simulink model "uz_mpc_6ph_sca"  (R2022b)
settings: Solver=FixedStepDiscrete  StartTime=0.0  StopTime=ST  RelTol=1e-3
InitFcn:
  | clear
  | clc
  | 
  | f_clock = 100e6;        % IP core clock freq in Hz
  | t_clock = 1/f_clock;    % IP core sample time in s
  | 
  | f_ADC =100e3;           % ADC interrupt freq in Hz
  | t_ADC = 1/f_ADC;        % ADC sample time in s
  | Ts = t_ADC;
  | 
  | % amplitude of sinusoidal signal sources
  | A = 0.1;
  | 
  | % machine parameters
  | Rs = 0.27;              % Phase resistance in Ohm
  | psi_pm = 0.19;          % PM flux linkage in Vs
  | Ld = 1.7e-3;            % d-inductance in H
  | Lq = 3.8e-3;            % q-inductance in H
  | Lx = 2.4e-3;            % x-inductance in H
  | Ly = 2.5e-3;            % y-inductance in H
  | p = 5;                  % pole pairs
  | 
  | VR = 400;               % Rated eff. line-line voltage in V
  | IR = 10/sqrt(2);             % Rated eff. phase current in A
  | % IR = 14.142;
  | nR = 3000;              % Rated mechanical speed in 1/min
  | 
  | % p.u. base units acc. to T.Geyer, Model predictive control of high power
  | % converters and industrial drives. Hoboken, NJ, USA: Wiley, 2016, Chapter 2.1.2
  | VB = sqrt(2/3)*VR;
  | IB = sqrt(2)*IR;
  | omegaB = nR*2*pi()/60*p;
  | ZB = VB/IB;
  | LB = ZB/omegaB;
  | SB = 3/2 *VB*IB;
  | psiB = VB/omegaB;
  | TB = psiB*IB;
  | 
  | %pre calculated constants - check results regarding fixd_type_constants!!!
  | Rs_over_ZB = Rs/ZB;
  | Ts_times_ZB_over_Ld = Ts*ZB/Ld;
  | Ts_times_ZB_over_Lq = Ts*ZB/Lq;
  | Ts_times_ZB_over_Lx = Ts*ZB/Lx;
  | Ts_times_ZB_over_Ly = Ts*ZB/Ly;
  | Ld_over_LB = Ld/LB;
  | Lq_over_LB = Lq/LB;
  | Ld_minus_Lq_over_LB = (Ld-Lq)/LB;
  | psi_pm_over_psiB = psi_pm/psiB;
  | 
  | % fixed-point data types
  | pu_fixdt_type = fixdt(1,18,15); % output data type of pu values
  | % fixdt_type_dq_currents = fixdt(1,27,16);
  | fixdt_type_dq_currents = fixdt(1,27,24);
  | fixdt_type_xy_currents = fixdt(1,18,11);
  | fixdt_type_dqxy_ref_currents = fixdt(1,18,15);
  | fixdt_type_dqxy_voltages = fixdt(1,27,24);
  | fixdt_type_angle = fixdt(1,24,20);
  | % fixdt_type_sin_cos = fixdt(1,18,16);
  | fixdt_type_sin_cos = fixdt(1,27,20);
  | fixdt_type_lambda = fixdt(0,18,17);
  | ... (+38 lines)
libraries: nesl_utility x44, fl_lib x41, simulink x23, ee_lib x12, hdlsllib x2, spsAlphaBetaZerotodq0Lib x1, batteryecm_lib x1
(part 2 of 4)

== system uz_mpc_6ph_sca/counter_f_sw_6ph ==
  note: To avoid unneccessary calcualtions, i divide by 24 on the ARM processor.
  note: Over AXI, 32 Bit are received.
      | However, only one Bit is used.
  note: 1 for one cycle if edge recognized
  note: Since i count now every On and Off Transition for each switch,
      |  i have to divide by 12*2 in order to get the switching frequency
      |  (after dividing by the time).
      | 12 comes from the 12 switches
      | 2 comes from that 1 ON-transition and 1 OFF-transition = 1 switching-cycle
  ss_in_0 : Inport
  ss_in_1 : Inport  Port=2
  ss_in_2 : Inport  Port=3
  ss_in_3 : Inport  Port=4
  ss_in_4 : Inport  Port=5
  ss_in_5 : Inport  Port=6
  ss_in_6 : Inport  Port=7
  ss_in_7 : Inport  Port=8
  ss_in_8 : Inport  Port=9
  ss_in_9 : Inport  Port=10
  ss_in_10 : Inport  Port=11
  ss_in_11 : Inport  Port=12
  bResetAXI : Inport  Port=13
  Count_f_sw : MATLAB Function  TreatAsAtomicUnit=on  VariantControl=(default)
  Detec_edge : Sum  Inputs=+-  AccumDataTypeStr=int8  OutDataTypeStr=int8
  Gain : Gain  Commented=on  Gain=1/(12*2)
  Mux : Mux  Inputs=6
  Mux1 : Mux  Inputs=6
  Mux2 : Mux  Inputs=2
  SS_Old : Delay  DelayLength=1
  Saturation : Saturate  UpperLimit=1  LowerLimit=0  OutMin=[0]  OutMax=[1]  OutDataTypeStr=fixdt(0,1)
  Scope : Scope  NumInputPorts=2
  delay : Delay  DelayLength=1
  reset_old2 : Delay  DelayLength=1
  reset_old_switch1 : Switch  Criteria=u2 ~= 0  SaturateOnIntegerOverflow=off  InputSameDT=off
  switchNumb_AXI : Outport  VectorParamsAs1DForOutWhenUnconnected=off
  switchNumb : Outport  Port=2  VectorParamsAs1DForOutWhenUnconnected=off
  wires:
  ss_in_9/1 -> Mux1/4
  ss_in_6/1 -> Mux1/1
  ss_in_10/1 -> Mux1/5
  ss_in_11/1 -> Mux1/6
  ss_in_8/1 -> Mux1/3
  ss_in_1/1 -> Mux/2
  ss_in_5/1 -> Mux/6
  Saturation/1 -> Count_f_sw/4(bReset), Scope/1
  ss_in_4/1 -> Mux/5
  Mux/1 -> Mux2/1
  ss_in_2/1 -> Mux/3
  ss_in_0/1 -> Mux/1
  Mux2/1 -> SS_Old/1, Count_f_sw/3(ss_v)
  delay/1 -> Count_f_sw/1(switchNumb)
  reset_old2/1 -> Detec_edge/2, reset_old_switch1/3
  Detec_edge/1 -> Saturation/1, reset_old_switch1/2  "1 for one cycle if edge recognized"
  Mux1/1 -> Mux2/2
  reset_old_switch1/1 -> reset_old2/1
  ss_in_7/1 -> Mux1/2
  bResetAXI/1 -> Scope/2, reset_old_switch1/1, Detec_edge/1
  ss_in_3/1 -> Mux/4
  SS_Old/1 -> Count_f_sw/2(ss_v_old)
  Count_f_sw/1(switchNumbOut) -> delay/1, switchNumb_AXI/1, switchNumb/1

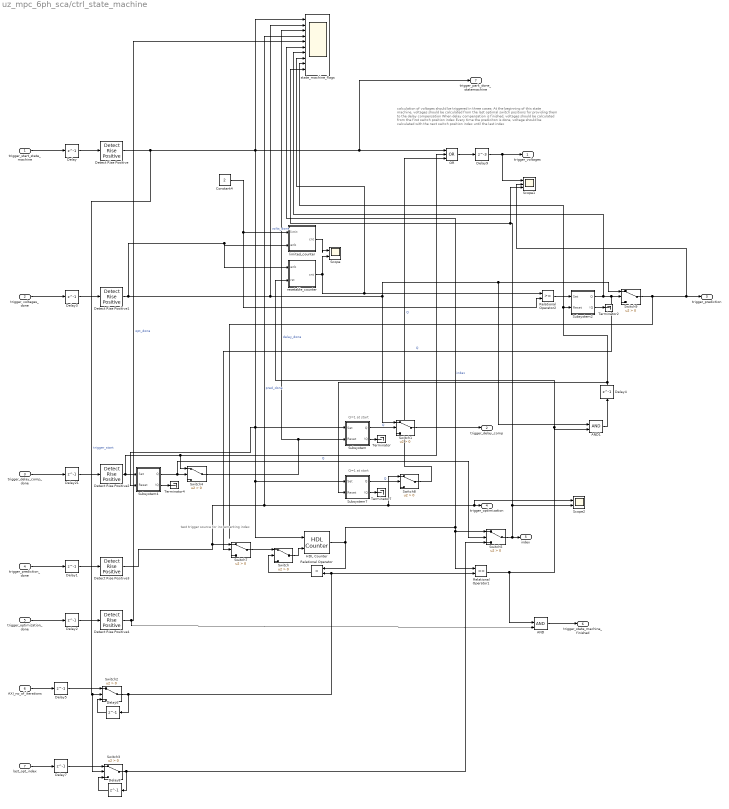
== system uz_mpc_6ph_sca/ctrl_state_machine ==
  note: test trigger source for incrementing index
  note: calculation of voltages should be triggered in three cases:
      |
      | At the beginning of this state machine, voltages should be calculated from the last optimal switch positions for providing them to the delay compensation
      | When delay compensation is finished, voltages should be calculated from the first switch position index
      | Every time the prediciton is done, voltage should be calculated with the next switch position index until the last index
  note: Q=1 at start
  note: Q=1 at start
  trigger_start_state_machine : Inport
  trigger_voltages_done : Inport  Port=2
  trigger_delay_comp_done : Inport  Port=3
  trigger_prediction_done : Inport  Port=4
  trigger_optimization_done : Inport  Port=5
  AXI_no_of_iterations : Inport  Port=6  OutDataTypeStr=uint32
  last_opt_index : Inport  Port=7  OutDataTypeStr=uint32
  AND : Logic  IconShape=distinctive  AllPortsSameDT=off  OutDataTypeStr=boolean
  AND1 : Logic  IconShape=distinctive  AllPortsSameDT=off  OutDataTypeStr=boolean
  Constant4 : Constant  Value=2  OutDataTypeStr=uint8  SampleTime=-1
  Delay{,1..8,21} (10 alike) : Delay  DelayLength=1
  Delay9 : Delay  DelayLength=3
  Detect Rise Positive{,1..4} (5 alike) : simulink/Logic and Bit Operations/Detect Rise Positive  vinit=0  OutDataTypeStr=boolean
  HDL Counter : hdlsllib/Sources/HDL Counter  CountType=Free running  CountInit=1  CountStep=1  CountMax=25  CountFromType=Initial value  CountFrom=1  CountResetPort=on  CountLoadPort=off  CountEnbPort=on  CountDirPort=off  CountHitOutputPort=off  CountDataType=Unsigned  CountWordLen=32  CountFracLen=0  CountSampTime=1
  OR : Logic  Operator=OR  Inputs=3  IconShape=distinctive  AllPortsSameDT=off  OutDataTypeStr=boolean
  Relational Operator : RelationalOperator  Operator=<  OutDataTypeStr=boolean  RndMeth=Simplest  InputSameDT=off
  Relational Operator1 : RelationalOperator  Operator===  OutDataTypeStr=boolean  RndMeth=Simplest  InputSameDT=off
  Relational Operator2 : RelationalOperator  OutDataTypeStr=boolean  RndMeth=Simplest  InputSameDT=off
  Scope : Scope  NumInputPorts=2
  Scope1 : Scope  NumInputPorts=3
  Scope2 : Scope  NumInputPorts=2
  Subsystem : Subsystem
  Subsystem2 : Subsystem
  Subsystem4 : Subsystem
  Subsystem7 : Subsystem
  Switch{,1..5,7..9} (9 alike) : Switch  Criteria=u2 > Threshold  SaturateOnIntegerOverflow=off  InputSameDT=off
  Terminator{,2,4,7} (4 alike) : Terminator
  limited_counter : Subsystem
  resetable_counter : Subsystem
  state_machine_flags : Scope  NumInputPorts=10
  trigger_voltages : Outport  VectorParamsAs1DForOutWhenUnconnected=off
  trigger_delay_comp : Outport  Port=2  VectorParamsAs1DForOutWhenUnconnected=off
  trigger_prediction : Outport  Port=3  VectorParamsAs1DForOutWhenUnconnected=off
  trigger_optimization : Outport  Port=4  VectorParamsAs1DForOutWhenUnconnected=off
  index : Outport  Port=5  VectorParamsAs1DForOutWhenUnconnected=off
  trigger_state_machine_finished : Outport  Port=6  VectorParamsAs1DForOutWhenUnconnected=off
  trigger_park_done_statemachine : Outport  Port=7  VectorParamsAs1DForOutWhenUnconnected=off
  wires:
  Switch2/1 -> Delay6/1, Relational Operator/2, Relational Operator1/2
  Relational Operator/1 -> Switch/2
  Detect Rise Positive/1 -> Switch3/2, Switch2/2, state_machine_flags/1, HDL Counter/1, Subsystem7/1(Set), Subsystem/1(Set), Subsystem4/2(Reset), trigger_park_done_statemachine/1, OR/1  "trigger_start"
  Subsystem/1(Q) -> Switch1/2  "Q"
  Subsystem/2(!Q) -> Terminator/1
  Switch1/1 -> trigger_delay_comp/1
  trigger_voltages_done/1 -> Delay3/1
  trigger_delay_comp_done/1 -> Delay21/1
  Delay21/1 -> Detect Rise Positive2/1
  Delay/1 -> Detect Rise Positive/1
  trigger_start_state_machine/1 -> Delay/1
  Delay2/1 -> Detect Rise Positive4/1
  trigger_optimization_done/1 -> Delay2/1
  Delay1/1 -> Detect Rise Positive3/1
  trigger_prediction_done/1 -> Delay1/1
  Subsystem4/1(Q) -> Switch5/2, Switch4/2  "Q"
  Subsystem4/2(!Q) -> Terminator4/1
  Detect Rise Positive2/1 -> OR/2, Switch4/1, Subsystem4/1(Set)
  Switch4/1 -> state_machine_flags/3, Subsystem/2(Reset)  "delay_done"
  Detect Rise Positive1/1 -> resetable_counter/1(enb), limited_counter/2(enb), state_machine_flags/2, AND1/1, Switch9/1, Switch1/1  "volts_done"
  Delay3/1 -> Detect Rise Positive1/1
  Subsystem2/2(!Q) -> Terminator2/1
  Subsystem2/1(Q) -> state_machine_flags/7, Switch7/2, Switch9/2  "Q"
  Constant4/1 -> Relational Operator2/2, limited_counter/1(limit)
  Relational Operator2/1 -> Subsystem2/1(Set)
  limited_counter/1(cnt) -> Scope/1
  Detect Rise Positive3/1 -> Switch7/1, state_machine_flags/4, Switch8/1, Scope2/1, trigger_optimization/1  "pred_done"
  Switch/1 -> HDL Counter/2
  HDL Counter/1 -> Switch5/1, Relational Operator1/1, state_machine_flags/6, Relational Operator/1  "index"
  Detect Rise Positive4/1 -> state_machine_flags/5, AND/2  "opt_done"
  Switch7/1 -> Switch/1
  resetable_counter/1(cnt) -> Scope/2, state_machine_flags/8, Relational Operator2/1
  Relational Operator1/1 -> AND1/2, resetable_counter/2(rst), AND/1
  Switch9/1 -> Scope1/2, trigger_prediction/1
  AND/1 -> trigger_state_machine_finished/1
  AND1/1 -> Delay4/1
  Delay4/1 -> state_machine_flags/9, Subsystem2/2(Reset), Subsystem7/2(Reset)
  Switch8/1 -> OR/3  "Q"
  Subsystem7/2(!Q) -> Terminator7/1
  Subsystem7/1(Q) -> Switch8/2  "Q"
  AXI_no_of_iterations/1 -> Delay5/1
  Delay5/1 -> Switch2/1
  Delay6/1 -> Switch2/3
  last_opt_index/1 -> Delay7/1
  Switch3/1 -> Switch5/3, Delay8/1
  Delay7/1 -> Switch3/1
  Delay8/1 -> Switch3/3
  Switch5/1 -> Scope1/3, state_machine_flags/10, Scope2/2, index/1
  OR/1 -> Delay9/1
  Delay9/1 -> Scope1/1, trigger_voltages/1

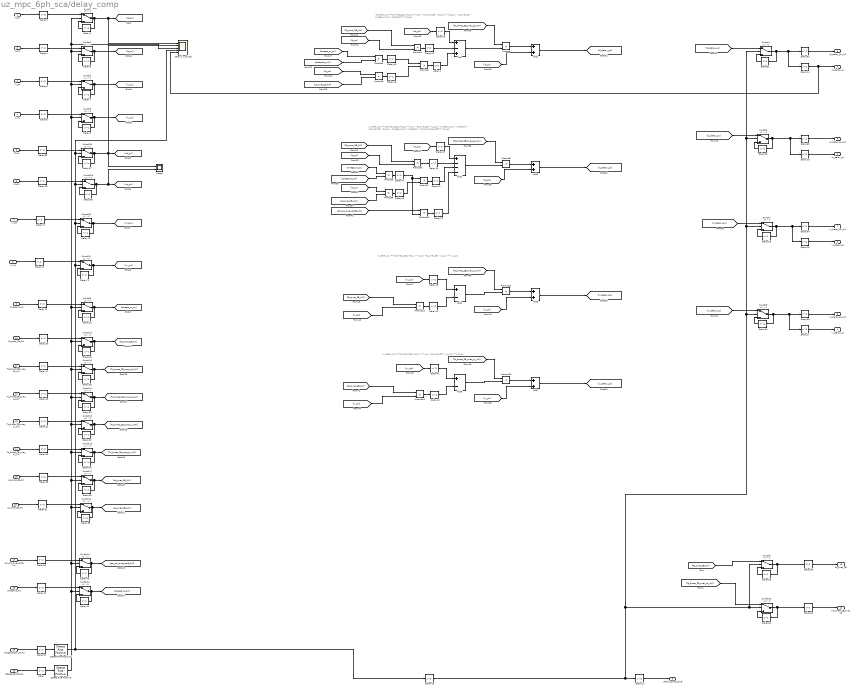
== system uz_mpc_6ph_sca/delay_comp ==
  note: iy_delay_pu = Ts_times_ZB_over_Ly *(vy_pu - Rs_over_ZB * iy_k_pu) + iy_k_pu
  note: ix_delay_pu = Ts_times_ZB_over_Lx *(vx_pu - Rs_over_ZB* ix_k_pu) + ix_k_pu
  note: iq_delay_pu = Ts_times_ZB_over_Lq *(vq_pu - Rs_over_ZB * iq_k_pu - omega_m_pu * polepairs * Ld_over_LB * id_k_pu - omega_m_pu * polepairs * psi_pm_over_psiB) + iq_k_pu
  note: id_delay_pu = Ts_times_ZB_over_Ld *(vd_pu - Rs_over_ZB * id_k_pu + iq_k_pu * Lq_over_LB * omega_m_pu * polepairs) + id_k_pu
  id_pu : Inport  OutDataTypeStr=fixdt_type_dq_currents
  iq_pu : Inport  Port=2  OutDataTypeStr=fixdt_type_dq_currents
  ix_pu : Inport  Port=3  OutDataTypeStr=fixdt_type_xy_currents
  iy_pu : Inport  Port=4  OutDataTypeStr=fixdt_type_xy_currents
  vd_pu : Inport  Port=5  OutDataTypeStr=fixdt_type_dqxy_voltages
  vq_pu : Inport  Port=6  OutDataTypeStr=fixdt_type_dqxy_voltages
  vx_pu : Inport  Port=7  OutDataTypeStr=fixdt_type_dqxy_voltages
  vy_pu : Inport  Port=8  OutDataTypeStr=fixdt_type_dqxy_voltages
  omega_m_pu : Inport  Port=9  OutDataTypeStr=fixdt_type_speed
  Rs_over_ZB_AXI : Inport  Port=10  OutDataTypeStr=fixdt_type_constants
  Ts_times_ZB_over_Ld_AXI : Inport  Port=11  OutDataTypeStr=fixdt_type_constants
  Ts_times_ZB_over_Lq_AXI : Inport  Port=12  OutDataTypeStr=fixdt_type_constants
  Ts_times_ZB_over_Lx_AXI : Inport  Port=13  OutDataTypeStr=fixdt_type_constants
  Ts_times_ZB_over_Ly_AXI : Inport  Port=14  OutDataTypeStr=fixdt_type_constants
  Ld_over_LB_AXI : Inport  Port=15  OutDataTypeStr=fixdt_type_constants
  Lq_over_LB_AXI : Inport  Port=16  OutDataTypeStr=fixdt_type_constants
  psi_pm_over_psiB_AXI : Inport  Port=17  OutDataTypeStr=fixdt_type_constants
  polepairs_AXI : Inport  Port=18  OutDataTypeStr=fixdt_type_polepairs
  trigger_delay_comp : Inport  Port=19
  trigger_park_done : Inport  Port=20
  Add : Sum  Inputs=+-+  AccumDataTypeStr=fixdt(1,27,16)
  Add{1,3,5,7} (4 alike) : Sum  AccumDataTypeStr=fixdt(1,27,24)
  Add2 : Sum  Inputs=+---  AccumDataTypeStr=fixdt(1,27,16)
  Add4 : Sum  Inputs=+-  AccumDataTypeStr=fixdt(1,27,16)
  Add6 : Sum  Inputs=+-  AccumDataTypeStr=fixdt(1,27,16)
  Delay{,2,4,6,8,10..12,14..20,23..25,27,29,31,33,35,37,39,41..43,49..50,56,59..60,62..66,71,73} (40 alike) : Delay
  Delay{1,3,5,7,9,13,21..22,26,28,30,32,34,36,38,40,44..48,51..55,57..58,61,70,72} (31 alike) : Delay  DelayLength=1
  Detect Rise Positive : simulink/Logic and Bit Operations/Detect Rise Positive  vinit=0  OutDataTypeStr=boolean
  Detect Rise Positive1 : simulink/Logic and Bit Operations/Detect Rise Positive  vinit=0  OutDataTypeStr=boolean
  Product{,1..2,4..7,9..14} (13 alike) : Product  OutDataTypeStr=fixdt(1,18,15)
  Product3 : Product  OutDataTypeStr=fixdt(1,27,16)
  Product8 : Product  OutDataTypeStr=fixdt(1,27,16)
  Scope : Scope  NumInputPorts=2
  Switch : Switch  Criteria=u2 > Threshold  OutDataTypeStr=fixdt_type_dq_currents  SaturateOnIntegerOverflow=off  InputSameDT=off
  Switch1 : Switch  Criteria=u2 > Threshold  OutDataTypeStr=fixdt_type_dq_currents  SaturateOnIntegerOverflow=off  InputSameDT=off
  Switch{4,6..10} (6 alike) : Switch  Criteria=u2 > Threshold  SaturateOnIntegerOverflow=off  InputSameDT=off
  Switch{12..19} (8 alike) : Switch  Criteria=u2 > Threshold  OutDataTypeStr=fixdt_type_constants  SaturateOnIntegerOverflow=off  InputSameDT=off
  Switch2 : Switch  Criteria=u2 > Threshold  OutDataTypeStr=fixdt_type_xy_currents  SaturateOnIntegerOverflow=off  InputSameDT=off
  Switch21 : Switch  Criteria=u2 > Threshold  OutDataTypeStr=fixdt_type_polepairs  SaturateOnIntegerOverflow=off  InputSameDT=off
  Switch{28..31} (4 alike) : Switch  Criteria=u2 > Threshold  OutDataTypeStr=fixdt_type_dqxy_voltages  SaturateOnIntegerOverflow=off  InputSameDT=off
  Switch3 : Switch  Criteria=u2 > Threshold  OutDataTypeStr=fixdt_type_xy_currents  SaturateOnIntegerOverflow=off  InputSameDT=off
  Switch5 : Switch  Criteria=u2 > Threshold  OutDataTypeStr=fixdt_type_speed  SaturateOnIntegerOverflow=off  InputSameDT=off
  delay_in_values : Scope  NumInputPorts=5
  id_delay_pu : Outport
  iq_delay_pu : Outport  Port=2
  ix_delay_pu : Outport  Port=3
  iy_delay_pu : Outport  Port=4
  id_delay_pu_AXI : Outport  Port=5
  iq_delay_pu_AXI : Outport  Port=6
  ix_delay_pu_AXI : Outport  Port=7
  iy_delay_pu_AXI : Outport  Port=8
  delay_comp_done : Outport  Port=9
  Rs_over_ZB : Outport  Port=10
  Ts_times_ZB_over_Ld : Outport  Port=11
  wires:
  Add5/1 -> [ix_delay_pu]
  Switch12/1 -> [Rs_over_ZB_AXI], Delay26/1
  Add3/1 -> [iq_delay_pu]
  Add1/1 -> [id_delay_pu]
  Add7/1 -> [iy_delay_pu]
  Delay5/1 -> Switch1/3
  Delay25/1 -> Switch12/1
  Delay59/1 -> Switch28/1
  Delay33/1 -> Switch16/1
  vx_pu/1 -> Delay71/1
  vd_pu/1 -> Delay59/1
  Switch15/1 -> [Ts_times_ZB_over_Lx_AXI], Delay32/1
  Ld_over_LB_AXI/1 -> Delay35/1
  Delay2/1 -> Switch/1
  Switch16/1 -> Delay34/1, [Ts_times_ZB_over_Ly_AXI]
  ix_pu/1 -> Delay6/1
  Delay38/1 -> Switch18/3
  Switch17/1 -> Delay36/1, [Ld_over_LB_AXI]
  Delay9/1 -> Switch3/3
  Switch13/1 -> [Ts_times_ZB_over_Ld_AXI], Delay28/1
  Delay/1 -> Detect Rise Positive/1
  Delay34/1 -> Switch16/3
  Delay44/1 -> Switch21/3
  Delay29/1 -> Switch14/1
  Delay8/1 -> Switch3/1
  Switch29/1 -> Scope/2, [vq_pu], Delay58/1
  Switch3/1 -> [iy_pu], Delay9/1
  polepairs_AXI/1 -> Delay43/1
  Delay72/1 -> Switch31/3
  Delay43/1 -> Switch21/1
  Switch14/1 -> [Ts_times_ZB_over_Lq_AXI], Delay30/1
  Delay28/1 -> Switch13/3
  psi_pm_over_psiB_AXI/1 -> Delay39/1
  Delay58/1 -> Switch29/3
  id_pu/1 -> Delay2/1
  Switch21/1 -> [polepairs_AXI], Delay44/1
  Switch/1 -> delay_in_values/1, [id_pu], Delay3/1
  Delay35/1 -> Switch17/1
  Delay31/1 -> Switch15/1
  Switch28/1 -> Scope/1, delay_in_values/2, [vd_pu], Delay57/1
  Ts_times_ZB_over_Ly_AXI/1 -> Delay33/1
  Delay7/1 -> Switch2/3
  Delay37/1 -> Switch18/1
  Delay4/1 -> Switch1/1
  Switch2/1 -> [ix_pu], Delay7/1
  Delay12/1 -> Switch5/1
  Delay73/1 -> Switch31/1
  Switch31/1 -> Delay72/1, [vy_pu]
  omega_m_pu/1 -> Delay12/1
  Delay6/1 -> Switch2/1
  Delay27/1 -> Switch13/1
  vq_pu/1 -> Delay60/1
  Switch5/1 -> [omega_m_pu], Delay13/1
  Lq_over_LB_AXI/1 -> Delay37/1
  iq_pu/1 -> Delay4/1
  iy_pu/1 -> Delay8/1
  vy_pu/1 -> Delay73/1
  Delay70/1 -> Switch30/3
  Delay60/1 -> Switch29/1
  Switch30/1 -> Delay70/1, [vx_pu]
  Ts_times_ZB_over_Lq_AXI/1 -> Delay29/1
  Delay3/1 -> Switch/3
  Switch18/1 -> Delay38/1, [Lq_over_LB_AXI]
  Delay26/1 -> Switch12/3
  Switch19/1 -> [psi_pm_over_psiB_AXI], Delay40/1
  Ts_times_ZB_over_Lx_AXI/1 -> Delay31/1
  Delay71/1 -> Switch30/1
  Switch1/1 -> [iq_pu], Delay5/1
  Ts_times_ZB_over_Ld_AXI/1 -> Delay27/1
  Delay57/1 -> Switch28/3
  Rs_over_ZB_AXI/1 -> Delay25/1
  Delay39/1 -> Switch19/1
  trigger_park_done/1 -> Delay/1
  Delay40/1 -> Switch19/3
  Delay13/1 -> Switch5/3
  Delay32/1 -> Switch15/3
  Delay36/1 -> Switch17/3
  Delay30/1 -> Switch14/3
  Delay11/1 -> delay_comp_done/1
  Switch8/1 -> Delay54/1, Delay17/1, Delay65/1
  Switch4/1 -> Delay51/1, Delay14/1, Delay62/1
  Delay63/1 -> iq_delay_pu_AXI/1
  Delay65/1 -> iy_delay_pu_AXI/1
  Delay64/1 -> ix_delay_pu_AXI/1
  Switch7/1 -> Delay53/1, Delay16/1, Delay64/1
  Delay62/1 -> id_delay_pu_AXI/1
  Delay15/1 -> iq_delay_pu/1
  Delay14/1 -> delay_in_values/5, id_delay_pu/1
  Delay16/1 -> ix_delay_pu/1
  Delay17/1 -> iy_delay_pu/1
  Add/1 -> Product/2
  [Ts_times_ZB_over_Ld_AXI] -> Product/1  "Ts_times_ZB_over_Ld"
  Product/1 -> Add1/1
  [id_pu] -> Add1/2  "id_k_pu"
  [Rs_over_ZB_AXI] -> Product1/1  "Rs_over_ZB"
  [id_pu] -> Product1/2  "id_k_pu"
  [iq_pu] -> Product3/1  "iq_k_pu"
  [Lq_over_LB_AXI] -> Product3/2  "Lq_over_LB"
  [omega_m_pu] -> Product4/1  "omega_m_pu"
  [polepairs_AXI] -> Product4/2  "polepairs"
  [Ts_times_ZB_over_Lq_AXI] -> Product5/1  "Ts_times_ZB_over_Lq"
  [iq_pu] -> Product6/2  "iq_k_pu"
  [Rs_over_ZB_AXI] -> Product6/1  "Rs_over_ZB"
  Add2/1 -> Product5/2
  [omega_m_pu] -> Product9/1  "omega_m_pu"
  [iq_pu] -> Add3/2  "iq_k_pu"
  [id_pu] -> Product8/1  "id_k_pu"
  [Ld_over_LB_AXI] -> Product8/2  "Ld_over_LB"
  [polepairs_AXI] -> Product9/2  "polepairs"
  Product5/1 -> Add3/1
  [psi_pm_over_psiB_AXI] -> Product10/1
  [Ts_times_ZB_over_Lx_AXI] -> Product11/1  "Ts_times_ZB_over_Lx"
  [ix_pu] -> Product12/2  "ix_k_pu"
  [Rs_over_ZB_AXI] -> Product12/1  "Rs_over_ZB"
  Add4/1 -> Product11/2
  [ix_pu] -> Add5/2  "ix_k_pu"
  Product11/1 -> Add5/1
  [Rs_over_ZB_AXI] -> Product14/1  "Rs_over_ZB"
  Add6/1 -> Product13/2
  [iy_pu] -> Add7/2  "iy_k_pu"
  [iy_pu] -> Product14/2  "iy_k_pu"
  [Ts_times_ZB_over_Ly_AXI] -> Product13/1  "Ts_times_ZB_over_Ly"
  Product13/1 -> Add7/1
  Product2/1 -> Delay1/1
  Product1/1 -> Delay10/1
  Delay10/1 -> Add/2
  Delay1/1 -> Add/3
  [vd_pu] -> Delay18/1  "vd_pu"
  Delay18/1 -> Add/1
  [vq_pu] -> Delay19/1  "vq_pu"
  Product7/1 -> Delay21/1
  Product10/1 -> Delay22/1
  Delay22/1 -> Add2/4
  Delay21/1 -> Add2/3
  Delay20/1 -> Add2/2
  Delay19/1 -> Add2/1
  Product6/1 -> Delay20/1
  [vx_pu] -> Delay23/1  "vx_pu"
  Delay23/1 -> Add4/1
  Product12/1 -> Delay24/1
  Delay24/1 -> Add4/2
  [vy_pu] -> Delay41/1  "vy_pu"
  Product14/1 -> Delay42/1
  Delay42/1 -> Add6/2
  Delay41/1 -> Add6/1
  Product4/1 -> Delay45/1
  Product3/1 -> Delay46/1
  Delay46/1 -> Product2/2
  Delay45/1 -> Product2/1
  Product9/1 -> Delay47/1
  Delay47/1 -> Product10/2, Product7/1
  Product8/1 -> Delay48/1
  Delay48/1 -> Product7/2
  trigger_delay_comp/1 -> Delay50/1
  Delay50/1 -> Detect Rise Positive1/1
  Detect Rise Positive/1 -> Switch21/2, Switch19/2, Switch18/2, Switch17/2, Switch16/2, Switch15/2, Switch14/2, Switch13/2, Switch12/2, Switch5/2, Switch3/2, Switch2/2, Switch1/2, Switch/2, delay_in_values/3
  Detect Rise Positive1/1 -> Delay49/1, delay_in_values/4, Switch28/2, Switch29/2, Switch30/2, Switch31/2  "delay_comp done"
  [id_delay_pu] -> Switch4/1
  Delay51/1 -> Switch4/3
  [iq_delay_pu] -> Switch6/1
  Switch6/1 -> Delay52/1, Delay15/1, Delay63/1
  Delay52/1 -> Switch6/3
  [ix_delay_pu] -> Switch7/1
  Delay53/1 -> Switch7/3
  Delay54/1 -> Switch8/3
  [iy_delay_pu] -> Switch8/1
  Switch9/1 -> Delay55/1, Delay56/1
  Delay55/1 -> Switch9/3
  [Rs_over_ZB_AXI] -> Switch9/1
  Delay49/1 -> Switch9/2, Switch10/2, Switch8/2, Switch7/2, Switch6/2, Switch4/2, Delay11/1
  Delay56/1 -> Rs_over_ZB/1
  Switch10/1 -> Delay61/1, Delay66/1
  Delay61/1 -> Switch10/3
  [Ts_times_ZB_over_Ld_AXI] -> Switch10/1
  Delay66/1 -> Ts_times_ZB_over_Ld/1

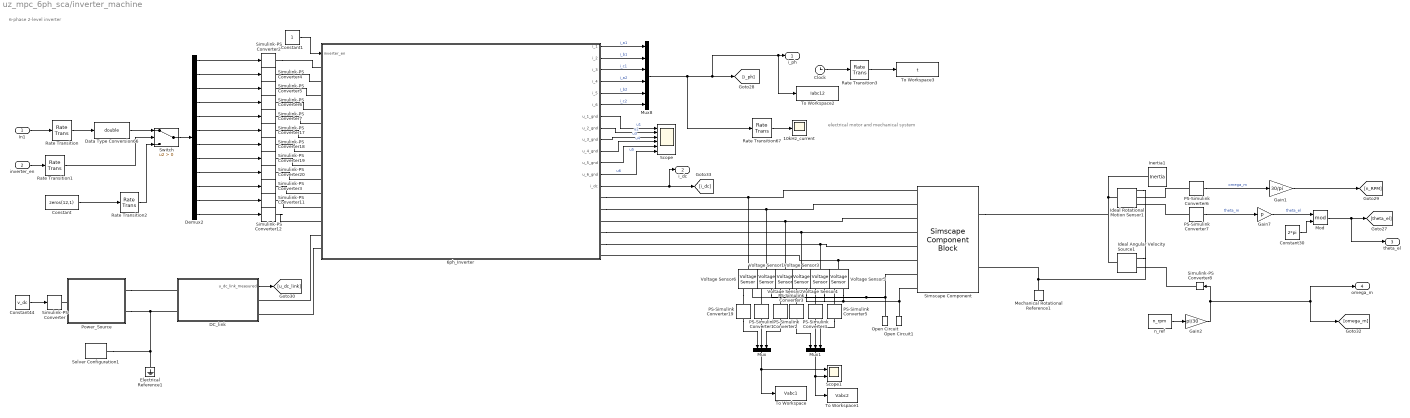
== system uz_mpc_6ph_sca/inverter_machine ==
  note: electrical motor and mechanical system
  note: 6-phase 2-level inverter
  In1 : Inport
  inverter_en : Inport  Port=2
  10kHz_current : Scope
  6ph_Inverter : Subsystem
  Clock : Clock
  Constant : Constant  Value=zeros(12,1)
  Constant1 : Constant  OutDataTypeStr=boolean
  Constant30 : Constant  Value=2*pi  SampleTime=-1
  Constant44 : Constant  Value=v_dc  SampleTime=-1
  DC_link : Subsystem
  Data Type Conversion66 : DataTypeConversion  OutDataTypeStr=double  SaturateOnIntegerOverflow=off  RndMeth=Floor
  Demux2 : Demux  Outputs=12
  Electrical Reference1 : fl_lib/Electrical/Electrical Elements/Electrical Reference
  Gain1 : Gain  Gain=30/pi
  Gain2 : Gain  Gain=pi/30
  Gain7 : Gain  Gain=p
  Ideal Angular Velocity Source1 : fl_lib/Mechanical/Mechanical Sources/Ideal Angular Velocity Source
  Ideal Rotational Motion Sensor1 : fl_lib/Mechanical/Mechanical Sensors/Ideal Rotational Motion Sensor  reference=foundation.enum.MeasurementReference.difference  acceleration_port=false  velocity_port=true  position_port=true  wrap_angle=simscape.enum.onoff.off  offset=0 deg
  Inertia1 : fl_lib/Mechanical/Rotational Elements/Inertia  inertia=J kg*m^2  num_ports=foundation.enum.numPorts2.one  w_specify=off  w_priority=High  w=0 rad/s  w_nominal_specify=off  w_nominal_unit=rad/s  w_nominal_value=1  t_specify=off  t_priority=None  t=0 N*m  t_nominal_specify=off  t_nominal_unit=N*m  t_nominal_value=1
  Mechanical Rotational Reference1 : fl_lib/Mechanical/Rotational Elements/Mechanical Rotational Reference
  Mod : Math  Operator=mod
  Mux : Mux  Inputs=3
  Mux1 : Mux  Inputs=3
  Mux8 : Mux  Inputs=6
  Open Circuit : fl_lib/Electrical/Electrical Elements/Open Circuit  v_specify=off  v_priority=None  v=0 V  v_nominal_specify=off  v_nominal_unit=V  v_nominal_value=1
  Open Circuit1 : fl_lib/Electrical/Electrical Elements/Open Circuit  v_specify=off  v_priority=None  v=0 V  v_nominal_specify=off  v_nominal_unit=V  v_nominal_value=1
  PS-Simulink Converter{1..5,19} (6 alike) : nesl_utility/PS-Simulink Converter  PhysicalDomain=network_engine_domain  SubClassName=ps_output  LeftPortType=input  RightPortType=output  PseudoPeriodic=off  Frequencies=[]  VectorFormat=1-D array  Unit=V  AffineConversion=off
  PS-Simulink Converter6 : nesl_utility/PS-Simulink Converter  PhysicalDomain=network_engine_domain  SubClassName=ps_output  LeftPortType=input  RightPortType=output  PseudoPeriodic=off  Frequencies=[]  VectorFormat=1-D array  Unit=1  AffineConversion=off
  PS-Simulink Converter7 : nesl_utility/PS-Simulink Converter  PhysicalDomain=network_engine_domain  SubClassName=ps_output  LeftPortType=input  RightPortType=output  PseudoPeriodic=off  Frequencies=[]  VectorFormat=1-D array  Unit=1  AffineConversion=off
  Power_Source : Subsystem
  Rate Transition{,1..3} (4 alike) : RateTransition  OutPortSampleTime=1e-6
  Rate Transition67 : RateTransition  OutPortSampleTime=0.0001
  Scope : Scope  NumInputPorts=6
  Scope1 : Scope  NumInputPorts=2
  Simscape Component : SimscapeComponentBlock  SourceFile=SixPhase_PMSM  ComponentPath=SixPhase_PMSM  ComponentVariants=SixPhase_PMSM  ComponentVariantNames=SixPhase_PMSM  ClassName=SixPhase_PMSM  SchemaVersion=1  Rs=Rs Ohm  Ld=Ld H  Lq=Lq H  Lx=Lx H  Ly=Ly H  psiPM=psi_pm Wb  np=p  theta_m_specify=off  theta_m_priority=None  theta_m=0 rad  theta_m_nominal_specify=off  theta_m_nominal_unit=rad  theta_m_nominal_value=1
      settings: CopyFcn=simscape.engine.sli.internal.componentblockcallback(gcbh,'COPY')  PreCopyFcn=simscape.engine.sli.internal.componentblockcallback(gcbh,'PRECOPY')  PreDeleteFcn=simscape.engine.sli.internal.componentblockcallback(gcbh,'PREDELETE')  InternalSimscapePortConfiguration="{\"Bottom\":[],\"Left\":[{\"id\":\"a1\",\"label\":\"a1\",\"type\":\"foundation.electrical.electrical\"},{\"id\":\"b1\",\"label\":\"b1\",\"type\":\"foundation.electrical.electrical\"},{\"id\":\"c1\",\"label\":\"c1\",\"type\":\"foundation.electrical.electrical\"},{\"id\":\"a2\",\"label\":\"a2\",\"type\":\"foundation.electrical.electrical\"},{\"id\":\"b2\",\"label\":\"b2\",\"type\":\"foundation.electrical.electrical\"},{\"id\":\"c2\",\"label\":\"c2\",\"type\":\"foundation.electrical.electrical\"},{\"id\":\"n1\",\"label\":\"n1\",\"type\":\"foundation.electrical.electrical\"},{\"id\":\"n2\",\"label\":\"n2\",\"type\":\"foundation.electrical.electrical\"}],\"Right\":[{\"id\":\"R\",\"label\":\"R\",\"type\":\"foundation.mechanical.rotational.rotational\"},{\"id\":\"C\",\"label\":\"C\",\"type\":\"foundation.mechanical.rotational.rotational\"}],\"Top\":[]}"
      mask Type: SixPhase_PMSM
  Simulink-PS Converter{,2..8,11..12,17..20} (14 alike) : nesl_utility/Simulink-PS Converter  PhysicalDomain=network_engine_domain  SubClassName=ps_input  LeftPortType=input  RightPortType=output  PseudoPeriodic=off  Frequencies=[]  NoiseDistribution=none  NoiseParameters=[]  Unit=1  AffineConversion=off  FilteringAndDerivatives=provide  SimscapeFilterOrder=1  InputFilterTimeConstant=0.001  UdotUserProvided=0
  Solver Configuration1 : nesl_utility/Solver Configuration  PhysicalDomain=network_engine_domain  SubClassName=solver  LeftPortType=input  RightPortType=generic  Tones=[]  Harmonics=[]  SimulateNoise=off  Profile=off  UseLocalSampling=off  EnableSwitchedLinearOptims=on  FrequencyDomain=off  UseCCode=off  RelTol=0.001  AbsTol=1e-06  MinStep=1e-09  ToWorkspace=off  RevertToSquareIcSolve=off  NumHomotopyIterations=100  PhasorMode=off  PhasorModeNumHarmonics=1  ConsistencySolver=NEWTON_FTOL  IndexReductionMethod=DerivativeReplacement  DoDC=off  ResidualTolerance=1e-09  ConsistencyTolSource=GLOBAL  ConsistencyAbsTol=0.001  ConsistencyRelTol=0.001  ConsistencyTolFactor=0.001  UseLocalSolver=on  LocalSolverChoice=NE_BACKWARD_EULER_ADVANCER  ResolveIndetEquations=on  FunctionEvalNumThread=1  LocalSolverSampleTime=1e-6  DoFixedCost=on  MaxNonlinIter=3  MaxModeIter=2  ComputeImpulses=off  ImpulseIterations=2  LinearAlgebra=Sparse  LinearAlgebraNumThread=0  EquationFormulation=NE_TIME_EF  DelaysMemoryBudget=1024  AutomaticFiltering=on  FilteringTimeConstant=0.001  PartitionStorageMethod=AS_NEEDED  PartitionMemoryBudget=1024  PartitionMethod=FAST
  Switch : Switch  Criteria=u2 > Threshold  SaturateOnIntegerOverflow=off  InputSameDT=off
  To Workspace : ToWorkspace  VariableName=Vabc1  SampleTime=-1
      settings: Save2DSignal=2-D array (concatenate along first dimension)
  To Workspace1 : ToWorkspace  VariableName=Vabc2  SampleTime=-1
      settings: Save2DSignal=2-D array (concatenate along first dimension)
  To Workspace2 : ToWorkspace  VariableName=Iabc12  SampleTime=-1
      settings: Save2DSignal=2-D array (concatenate along first dimension)
  To Workspace3 : ToWorkspace  VariableName=t  SampleTime=-1
      settings: Save2DSignal=2-D array (concatenate along first dimension)
  Voltage Sensor{1..6} (6 alike) : fl_lib/Electrical/Electrical Sensors/Voltage Sensor
  n_ref : Constant  Value=n_rpm  SampleTime=-1
  i_ph : Outport
  i_dc : Outport  Port=2
  theta_el : Outport  Port=3
  omega_m : Outport  Port=4
  wires:
  Mux8/1 -> Rate Transition67/1, To Workspace2/1, i_ph/1, [i_ph]
  Demux2/11 -> Simulink-PS Converter11/1
  Gain2/1 -> [omega_m], omega_m/1, Simulink-PS Converter8/1
  Gain7/1 -> Mod/1  "theta_el"
  6ph_Inverter/3(i_3) -> Mux8/3  "i_c1"
  6ph_Inverter/5(i_5) -> Mux8/5  "i_b2"
  PS-Simulink Converter6/1 -> Gain1/1  "omega_m"
  Gain1/1 -> [n_RPM]
  Demux2/6 -> Simulink-PS Converter17/1
  Demux2/5 -> Simulink-PS Converter7/1
  6ph_Inverter/13(i_dc) -> i_dc/1, [i_dc]
  PS-Simulink Converter7/1 -> Gain7/1  "theta_m"
  Data Type Conversion66/1 -> Switch/1
  Mod/1 -> theta_el/1, [theta_el]
  6ph_Inverter/2(i_2) -> Mux8/2  "i_b1"
  DC_link/1(u_dc_link_measured) -> [u_dc_link]
  In1/1 -> Rate Transition/1
  Demux2/12 -> Simulink-PS Converter12/1
  Demux2/4 -> Simulink-PS Converter6/1
  Demux2/9 -> Simulink-PS Converter20/1
  Constant30/1 -> Mod/2
  Demux2/7 -> Simulink-PS Converter18/1
  6ph_Inverter/1(i_1) -> Mux8/1  "i_a1"
  Constant44/1 -> Simulink-PS Converter/1
  Demux2/1 -> Simulink-PS Converter2/1
  Demux2/2 -> Simulink-PS Converter4/1
  Demux2/10 -> Simulink-PS Converter3/1
  6ph_Inverter/4(i_4) -> Mux8/4  "i_a2"
  Demux2/8 -> Simulink-PS Converter19/1
  Rate Transition/1 -> Data Type Conversion66/1
  6ph_Inverter/6(i_6) -> Mux8/6  "i_c2"
  n_ref/1 -> Gain2/1
  Demux2/3 -> Simulink-PS Converter5/1
  Rate Transition67/1 -> 10kHz_current/1
  inverter_en/1 -> Rate Transition1/1
  Switch/1 -> Demux2/1
  Constant/1 -> Rate Transition2/1
  Constant1/1 -> 6ph_Inverter/1(inverter_en)
  Rate Transition1/1 -> Switch/2
  Rate Transition2/1 -> Switch/3
  6ph_Inverter/7(u_1_gnd) -> Scope/1  "u1"
  6ph_Inverter/8(u_2_gnd) -> Scope/2  "u2"
  6ph_Inverter/9(u_3_gnd) -> Scope/3  "u3"
  6ph_Inverter/10(u_4_gnd) -> Scope/4  "u4"
  6ph_Inverter/11(u_5_gnd) -> Scope/5  "u5"
  6ph_Inverter/12(u_6_gnd) -> Scope/6  "u6"
  PS-Simulink Converter19/1 -> Mux/1
  PS-Simulink Converter1/1 -> Mux/2
  PS-Simulink Converter2/1 -> Mux/3
  PS-Simulink Converter3/1 -> Mux1/1
  PS-Simulink Converter4/1 -> Mux1/2
  PS-Simulink Converter5/1 -> Mux1/3
  Mux/1 -> To Workspace/1, Scope1/1
  Mux1/1 -> To Workspace1/1, Scope1/2
  Clock/1 -> Rate Transition3/1
  Rate Transition3/1 -> To Workspace3/1
  connections:
  Simulink-PS Converter6/RConn1 -- 6ph_Inverter/LConn4
  PS-Simulink Converter6/LConn1 -- Ideal Rotational Motion Sensor1/RConn2
  Electrical Reference1/LConn1 -- DC_link/LConn2 -- Power_Source/RConn2 -- Solver Configuration1/RConn1
  Simscape Component/LConn6 -- 6ph_Inverter/RConn6 -- Voltage Sensor5/LConn1
  Ideal Rotational Motion Sensor1/LConn1 -- Ideal Angular Velocity Source1/LConn1 -- Simscape Component/RConn1 -- Inertia1/LConn1
  Mechanical Rotational Reference1/LConn1 -- Simscape Component/RConn2 -- Ideal Rotational Motion Sensor1/RConn1 -- Ideal Angular Velocity Source1/RConn2
  Simulink-PS Converter3/RConn1 -- 6ph_Inverter/LConn10
  Simulink-PS Converter11/RConn1 -- 6ph_Inverter/LConn11
  Simscape Component/LConn3 -- Voltage Sensor2/LConn1 -- 6ph_Inverter/RConn3
  6ph_Inverter/LConn14 -- DC_link/RConn2
  Simulink-PS Converter12/RConn1 -- 6ph_Inverter/LConn12
  6ph_Inverter/RConn4 -- Simscape Component/LConn4 -- Voltage Sensor3/LConn1
  Simulink-PS Converter17/RConn1 -- 6ph_Inverter/LConn6
  Simscape Component/LConn7 -- Voltage Sensor2/RConn2 -- Voltage Sensor1/RConn2 -- Voltage Sensor6/RConn2 -- Open Circuit/LConn1
  Simulink-PS Converter7/RConn1 -- 6ph_Inverter/LConn5
  Simscape Component/LConn8 -- Voltage Sensor3/RConn2 -- Voltage Sensor4/RConn2 -- Voltage Sensor5/RConn2 -- Open Circuit1/LConn1
  6ph_Inverter/RConn2 -- Simscape Component/LConn2 -- Voltage Sensor1/LConn1
  Simulink-PS Converter/RConn1 -- Power_Source/LConn1
  Simulink-PS Converter19/RConn1 -- 6ph_Inverter/LConn8
  PS-Simulink Converter7/LConn1 -- Ideal Rotational Motion Sensor1/RConn3
  Simulink-PS Converter5/RConn1 -- 6ph_Inverter/LConn3
  6ph_Inverter/RConn5 -- Simscape Component/LConn5 -- Voltage Sensor4/LConn1
  Simulink-PS Converter4/RConn1 -- 6ph_Inverter/LConn2
  Simulink-PS Converter8/RConn1 -- Ideal Angular Velocity Source1/RConn1
  Power_Source/RConn1 -- DC_link/LConn1
  6ph_Inverter/LConn13 -- DC_link/RConn1
  6ph_Inverter/RConn1 -- Simscape Component/LConn1 -- Voltage Sensor6/LConn1
  Simulink-PS Converter18/RConn1 -- 6ph_Inverter/LConn7
  Simulink-PS Converter2/RConn1 -- 6ph_Inverter/LConn1
  Simulink-PS Converter20/RConn1 -- 6ph_Inverter/LConn9
  Voltage Sensor6/RConn1 -- PS-Simulink Converter19/LConn1
  PS-Simulink Converter1/LConn1 -- Voltage Sensor1/RConn1
  PS-Simulink Converter2/LConn1 -- Voltage Sensor2/RConn1
  PS-Simulink Converter3/LConn1 -- Voltage Sensor3/RConn1
  PS-Simulink Converter4/LConn1 -- Voltage Sensor4/RConn1
  PS-Simulink Converter5/LConn1 -- Voltage Sensor5/RConn1

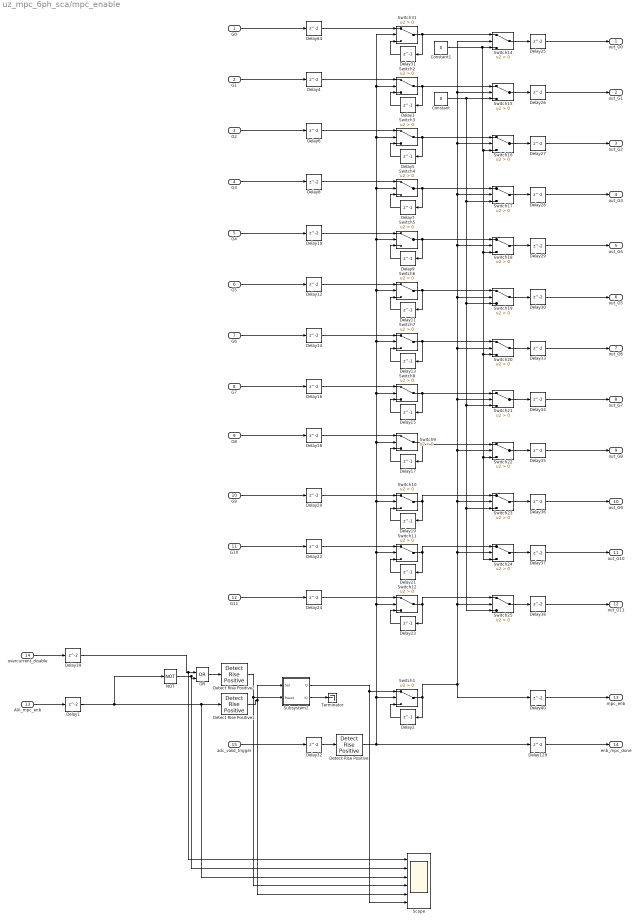
== system uz_mpc_6ph_sca/mpc_enable ==
  G0 : Inport
  G1 : Inport  Port=2
  G2 : Inport  Port=3
  G3 : Inport  Port=4
  G4 : Inport  Port=5
  G5 : Inport  Port=6
  G6 : Inport  Port=7
  G7 : Inport  Port=8
  G8 : Inport  Port=9
  G9 : Inport  Port=10
  G10 : Inport  Port=11
  G11 : Inport  Port=12
  AXI_mpc_enb : Inport  Port=13
  overcurrent_disable : Inport  Port=14
  adc_valid_trigger : Inport  Port=15  OutDataTypeStr=boolean
  Constant : Constant  Value=0  OutDataTypeStr=boolean  SampleTime=-1
  Constant1 : Constant  Value=0  OutDataTypeStr=boolean  SampleTime=-1
  Delay{1,4,6,8,10,12,14,16,18,20,22,24..30,32..40,64,129} (29 alike) : Delay
  Delay{2..3,5,7,9,11,13,15,17,19,21,23,31} (13 alike) : Delay  DelayLength=1
  Detect Rise Positive : simulink/Logic and Bit Operations/Detect Rise Positive  vinit=0  OutDataTypeStr=boolean
  Detect Rise Positive1 : simulink/Logic and Bit Operations/Detect Rise Positive  vinit=0  OutDataTypeStr=boolean
  Detect Rise Positive2 : simulink/Logic and Bit Operations/Detect Rise Positive  vinit=0  OutDataTypeStr=boolean
  NOT : Logic  Operator=NOT  IconShape=distinctive  AllPortsSameDT=off  OutDataTypeStr=boolean
  OR : Logic  Operator=OR  IconShape=distinctive  AllPortsSameDT=off  OutDataTypeStr=boolean
  Scope : Scope  NumInputPorts=6
  Subsystem2 : Subsystem
  Switch{1..12,14..25,31} (25 alike) : Switch  Criteria=u2 > Threshold  SaturateOnIntegerOverflow=off  InputSameDT=off
  Terminator : Terminator
  out_G0 : Outport
  out_G1 : Outport  Port=2
  out_G2 : Outport  Port=3
  out_G3 : Outport  Port=4
  out_G4 : Outport  Port=5
  out_G5 : Outport  Port=6
  out_G6 : Outport  Port=7
  out_G7 : Outport  Port=8
  out_G8 : Outport  Port=9
  out_G9 : Outport  Port=10
  out_G10 : Outport  Port=11
  out_G11 : Outport  Port=12
  mpc_enb : Outport  Port=13  OutDataTypeStr=boolean  LockScale=on
  enb_mpc_done : Outport  Port=14  OutDataTypeStr=boolean  LockScale=on
  wires:
  adc_valid_trigger/1 -> Delay32/1
  G0/1 -> Delay64/1
  Delay129/1 -> enb_mpc_done/1
  Delay64/1 -> Switch31/1
  Delay32/1 -> Detect Rise Positive/1
  Switch31/1 -> Switch14/1, Delay31/1
  Delay31/1 -> Switch31/3
  AXI_mpc_enb/1 -> Delay1/1
  Delay2/1 -> Switch1/3
  Delay3/1 -> Switch2/3
  Switch2/1 -> Switch15/1, Delay3/1
  Delay4/1 -> Switch2/1
  G1/1 -> Delay4/1
  Detect Rise Positive/1 -> Delay129/1, Switch31/2, Switch2/2, Switch3/2, Switch4/2, Switch5/2, Switch6/2, Switch7/2, Switch8/2, Switch9/2, Switch10/2, Switch11/2, Switch12/2, Switch1/2
  Delay5/1 -> Switch3/3
  Switch3/1 -> Switch16/1, Delay5/1
  Delay6/1 -> Switch3/1
  G2/1 -> Delay6/1
  Delay7/1 -> Switch4/3
  Switch4/1 -> Switch17/1, Delay7/1
  Delay8/1 -> Switch4/1
  G3/1 -> Delay8/1
  Delay9/1 -> Switch5/3
  Switch5/1 -> Switch18/1, Delay9/1
  Delay10/1 -> Switch5/1
  G4/1 -> Delay10/1
  Delay11/1 -> Switch6/3
  Switch6/1 -> Switch19/1, Delay11/1
  Delay12/1 -> Switch6/1
  G5/1 -> Delay12/1
  Delay13/1 -> Switch7/3
  Switch7/1 -> Switch20/1, Delay13/1
  Delay14/1 -> Switch7/1
  G6/1 -> Delay14/1
  Delay15/1 -> Switch8/3
  Switch8/1 -> Switch21/1, Delay15/1
  Delay16/1 -> Switch8/1
  G7/1 -> Delay16/1
  Delay17/1 -> Switch9/3
  Switch9/1 -> Switch22/1, Delay17/1
  Delay18/1 -> Switch9/1
  G8/1 -> Delay18/1
  Delay19/1 -> Switch10/3
  Switch10/1 -> Delay19/1, Switch23/1
  Delay20/1 -> Switch10/1
  G9/1 -> Delay20/1
  Delay21/1 -> Switch11/3
  Switch11/1 -> Switch24/1, Delay21/1
  Delay22/1 -> Switch11/1
  G10/1 -> Delay22/1
  Delay23/1 -> Switch12/3
  Switch12/1 -> Switch25/1, Delay23/1
  Delay24/1 -> Switch12/1
  G11/1 -> Delay24/1
  Switch14/1 -> Delay25/1
  Delay25/1 -> out_G0/1
  Constant1/1 -> Switch24/3, Switch22/3, Switch20/3, Switch18/3, Switch16/3, Switch14/3
  Switch15/1 -> Delay26/1
  Delay26/1 -> out_G1/1
  Switch1/1 -> Delay40/1, Switch25/2, Switch24/2, Switch23/2, Switch22/2, Switch21/2, Switch20/2, Switch19/2, Switch18/2, Switch17/2, Switch16/2, Switch15/2, Switch14/2, Delay2/1
  Switch16/1 -> Delay27/1
  Delay28/1 -> out_G3/1
  Switch17/1 -> Delay28/1
  Delay27/1 -> out_G2/1
  Delay29/1 -> out_G4/1
  Switch19/1 -> Delay30/1
  Switch18/1 -> Delay29/1
  Delay30/1 -> out_G5/1
  Switch22/1 -> Delay35/1
  Switch20/1 -> Delay33/1
  Delay35/1 -> out_G8/1
  Switch23/1 -> Delay36/1
  Delay33/1 -> out_G6/1
  Delay36/1 -> out_G9/1
  Delay38/1 -> out_G11/1
  Switch25/1 -> Delay38/1
  Switch24/1 -> Delay37/1
  Delay34/1 -> out_G7/1
  Delay37/1 -> out_G10/1
  Switch21/1 -> Delay34/1
  Constant/1 -> Switch25/3, Switch23/3, Switch21/3, Switch19/3, Switch17/3, Switch15/3
  Subsystem2/1(Q) -> Scope/6, Switch1/1
  Detect Rise Positive1/1 -> Subsystem2/1(Set), Scope/5
  Detect Rise Positive2/1 -> Subsystem2/2(Reset), Scope/4
  OR/1 -> Detect Rise Positive2/1
  NOT/1 -> Scope/2, OR/2
  overcurrent_disable/1 -> Delay39/1
  Delay39/1 -> Scope/1, OR/1
  Delay1/1 -> Scope/3, Detect Rise Positive1/1, NOT/1
  Delay40/1 -> mpc_enb/1
  Subsystem2/2(!Q) -> Terminator/1

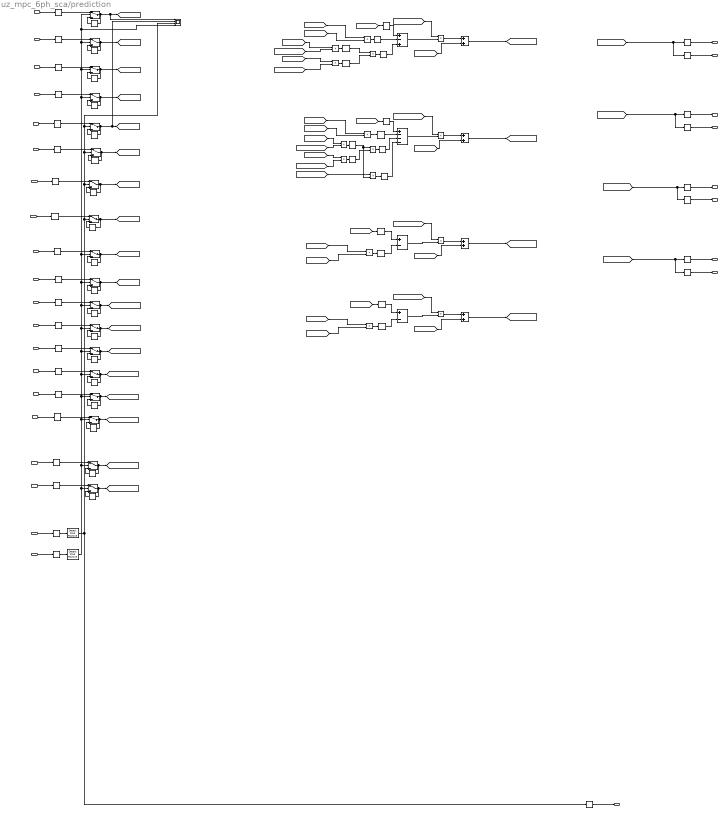
== system uz_mpc_6ph_sca/prediction ==
  note: voltages are triggered every iteration
  note: iy_delay_pu = Ts_times_ZB_over_Ly *(vy_pu - Rs_over_ZB * iy_k_pu) + iy_k_pu
  note: ix_delay_pu = Ts_times_ZB_over_Lx *(vx_pu - Rs_over_ZB* ix_k_pu) + ix_k_pu
  note: iq_delay_pu = Ts_times_ZB_over_Lq *(vq_pu - Rs_over_ZB * iq_k_pu - omega_m_pu * polepairs * Ld_over_LB * id_k_pu - omega_m_pu * polepairs * psi_pm_over_psiB) + iq_k_pu
  note: id_delay_pu = Ts_times_ZB_over_Ld *(vd_pu - Rs_over_ZB * id_k_pu + iq_k_pu * Lq_over_LB * omega_m_pu * polepairs) + id_k_pu
  id_delay_pu : Inport  OutDataTypeStr=fixdt_type_dq_currents
  iq_delay_pu : Inport  Port=2  OutDataTypeStr=fixdt_type_dq_currents
  ix_delay_pu : Inport  Port=3  OutDataTypeStr=fixdt_type_dq_currents
  iy_delay_pu : Inport  Port=4  OutDataTypeStr=fixdt_type_dq_currents
  vd_pu : Inport  Port=5  OutDataTypeStr=fixdt_type_dqxy_voltages
  vq_pu : Inport  Port=6  OutDataTypeStr=fixdt_type_dqxy_voltages
  vx_pu : Inport  Port=7  OutDataTypeStr=fixdt_type_dqxy_voltages
  vy_pu : Inport  Port=8  OutDataTypeStr=fixdt_type_dqxy_voltages
  omega_m_pu : Inport  Port=9  OutDataTypeStr=fixdt_type_speed
  Rs_over_ZB_AXI : Inport  Port=10  OutDataTypeStr=fixdt_type_constants
  Ts_times_ZB_over_Ld_AXI : Inport  Port=11  OutDataTypeStr=fixdt_type_constants
  Ts_times_ZB_over_Lq_AXI : Inport  Port=12  OutDataTypeStr=fixdt_type_constants
  Ts_times_ZB_over_Lx_AXI : Inport  Port=13  OutDataTypeStr=fixdt_type_constants
  Ts_times_ZB_over_Ly_AXI : Inport  Port=14  OutDataTypeStr=fixdt_type_constants
  Ld_over_LB_AXI : Inport  Port=15  OutDataTypeStr=fixdt_type_constants
  Lq_over_LB_AXI : Inport  Port=16  OutDataTypeStr=fixdt_type_constants
  psi_pm_over_psiB_AXI : Inport  Port=17  OutDataTypeStr=fixdt_type_constants
  polepairs_AXI : Inport  Port=18  OutDataTypeStr=fixdt_type_polepairs
  trigger_prediction : Inport  Port=19
  trigger_delay_comp_done : Inport  Port=20
  Add : Sum  Inputs=+-+  AccumDataTypeStr=fixdt(1,27,16)
  Add{1,3,5,7} (4 alike) : Sum  AccumDataTypeStr=fixdt(1,27,24)
  Add2 : Sum  Inputs=+---  AccumDataTypeStr=fixdt(1,27,16)
  Add4 : Sum  Inputs=+-  AccumDataTypeStr=fixdt(1,27,16)
  Add6 : Sum  Inputs=+-  AccumDataTypeStr=fixdt(1,27,16)
  Delay{,2,4,6,8,11..12,14..17,25,27,29,31,33,35,37,39,43,50,59..60,62..65,71,73} (29 alike) : Delay
  Delay{1,3,5,7,9..10,13,18..24,26,28,30,32,34,36,38,40..42,44..48,57..58,70,72} (33 alike) : Delay  DelayLength=1
  Detect Rise Positive : simulink/Logic and Bit Operations/Detect Rise Positive  vinit=0  OutDataTypeStr=boolean
  Detect Rise Positive1 : simulink/Logic and Bit Operations/Detect Rise Positive  vinit=0  OutDataTypeStr=boolean
  Product{,1..2,4..7,9..14} (13 alike) : Product  OutDataTypeStr=fixdt(1,18,15)
  Product3 : Product  OutDataTypeStr=fixdt(1,27,16)
  Product8 : Product  OutDataTypeStr=fixdt(1,27,16)
  Scope : Scope  NumInputPorts=4
  Switch{,1..3} (4 alike) : Switch  Criteria=u2 > Threshold  OutDataTypeStr=fixdt_type_dq_currents  SaturateOnIntegerOverflow=off  InputSameDT=off
  Switch{12..19} (8 alike) : Switch  Criteria=u2 > Threshold  OutDataTypeStr=fixdt_type_constants  SaturateOnIntegerOverflow=off  InputSameDT=off
  Switch21 : Switch  Criteria=u2 > Threshold  OutDataTypeStr=fixdt_type_polepairs  SaturateOnIntegerOverflow=off  InputSameDT=off
  Switch{28..31} (4 alike) : Switch  Criteria=u2 > Threshold  OutDataTypeStr=fixdt_type_dqxy_voltages  SaturateOnIntegerOverflow=off  InputSameDT=off
  Switch5 : Switch  Criteria=u2 > Threshold  OutDataTypeStr=fixdt_type_speed  SaturateOnIntegerOverflow=off  InputSameDT=off
  id_pred_pu : Outport
  iq_pred_pu : Outport  Port=2
  ix_pred_pu : Outport  Port=3
  iy_pred_pu : Outport  Port=4
  id_pred_pu_AXI : Outport  Port=5
  iq_pred_pu_AXI : Outport  Port=6
  ix_pred_pu_AXI : Outport  Port=7
  iy_pred_pu_AXI : Outport  Port=8
  prediction_done : Outport  Port=9
  wires:
  Add5/1 -> [ix_delay_pu]
  Switch12/1 -> [Rs_over_ZB_AXI], Delay26/1
  Add3/1 -> [iq_delay_pu]
  Add1/1 -> [id_delay_pu]
  Add7/1 -> [iy_delay_pu]
  Delay5/1 -> Switch1/3
  Delay25/1 -> Switch12/1
  Delay59/1 -> Switch28/1
  Delay33/1 -> Switch16/1
  vx_pu/1 -> Delay71/1
  vd_pu/1 -> Delay59/1
  Switch15/1 -> [Ts_times_ZB_over_Lx_AXI], Delay32/1
  Ld_over_LB_AXI/1 -> Delay35/1
  Delay2/1 -> Switch/1
  Switch16/1 -> Delay34/1, [Ts_times_ZB_over_Ly_AXI]
  ix_delay_pu/1 -> Delay6/1
  Delay38/1 -> Switch18/3
  Switch17/1 -> Delay36/1, [Ld_over_LB_AXI]
  Delay9/1 -> Switch3/3
  Switch13/1 -> [Ts_times_ZB_over_Ld_AXI], Delay28/1
  Delay/1 -> Detect Rise Positive/1
  Delay34/1 -> Switch16/3
  Delay44/1 -> Switch21/3
  Delay29/1 -> Switch14/1
  Delay8/1 -> Switch3/1
  Switch29/1 -> [vq_pu], Delay58/1
  Switch3/1 -> [iy_pu], Delay9/1
  polepairs_AXI/1 -> Delay43/1
  Delay72/1 -> Switch31/3
  Delay43/1 -> Switch21/1
  Switch14/1 -> [Ts_times_ZB_over_Lq_AXI], Delay30/1
  Delay28/1 -> Switch13/3
  psi_pm_over_psiB_AXI/1 -> Delay39/1
  Delay58/1 -> Switch29/3
  id_delay_pu/1 -> Delay2/1
  Switch21/1 -> [polepairs_AXI], Delay44/1
  Switch/1 -> Scope/1, [id_pu], Delay3/1
  Delay35/1 -> Switch17/1
  Delay31/1 -> Switch15/1
  Switch28/1 -> Scope/2, [vd_pu], Delay57/1
  Ts_times_ZB_over_Ly_AXI/1 -> Delay33/1
  Delay7/1 -> Switch2/3
  Delay37/1 -> Switch18/1
  Delay4/1 -> Switch1/1
  Switch2/1 -> [ix_pu], Delay7/1
  Delay12/1 -> Switch5/1
  Delay73/1 -> Switch31/1
  Switch31/1 -> Delay72/1, [vy_pu]
  omega_m_pu/1 -> Delay12/1
  Delay6/1 -> Switch2/1
  Delay27/1 -> Switch13/1
  vq_pu/1 -> Delay60/1
  Switch5/1 -> [omega_m_pu], Delay13/1
  Lq_over_LB_AXI/1 -> Delay37/1
  iq_delay_pu/1 -> Delay4/1
  iy_delay_pu/1 -> Delay8/1
  vy_pu/1 -> Delay73/1
  Delay70/1 -> Switch30/3
  Delay60/1 -> Switch29/1
  Switch30/1 -> Delay70/1, [vx_pu]
  Ts_times_ZB_over_Lq_AXI/1 -> Delay29/1
  Delay3/1 -> Switch/3
  Switch18/1 -> Delay38/1, [Lq_over_LB_AXI]
  Delay26/1 -> Switch12/3
  Switch19/1 -> [psi_pm_over_psiB_AXI], Delay40/1
  Ts_times_ZB_over_Lx_AXI/1 -> Delay31/1
  Delay71/1 -> Switch30/1
  Switch1/1 -> [iq_pu], Delay5/1
  Ts_times_ZB_over_Ld_AXI/1 -> Delay27/1
  Delay57/1 -> Switch28/3
  Rs_over_ZB_AXI/1 -> Delay25/1
  Delay39/1 -> Switch19/1
  trigger_delay_comp_done/1 -> Delay/1
  Delay40/1 -> Switch19/3
  Delay13/1 -> Switch5/3
  Delay32/1 -> Switch15/3
  Delay36/1 -> Switch17/3
  Delay30/1 -> Switch14/3
  Delay11/1 -> prediction_done/1
  [iy_delay_pu] -> Delay17/1, Delay65/1
  [iq_delay_pu] -> Delay15/1, Delay63/1
  [id_delay_pu] -> Delay14/1, Delay62/1
  Delay63/1 -> iq_pred_pu_AXI/1
  Delay65/1 -> iy_pred_pu_AXI/1
  Delay64/1 -> ix_pred_pu_AXI/1
  [ix_delay_pu] -> Delay16/1, Delay64/1
  Delay62/1 -> id_pred_pu_AXI/1
  Delay15/1 -> iq_pred_pu/1
  Delay14/1 -> id_pred_pu/1
  Delay16/1 -> ix_pred_pu/1
  Delay17/1 -> iy_pred_pu/1
  Add/1 -> Product/2
  [Ts_times_ZB_over_Ld_AXI] -> Product/1  "Ts_times_ZB_over_Ld"
  Product/1 -> Add1/1
  [id_pu] -> Add1/2  "id_k_pu"
  [Rs_over_ZB_AXI] -> Product1/1  "Rs_over_ZB"
  [id_pu] -> Product1/2  "id_k_pu"
  [iq_pu] -> Product3/1  "iq_k_pu"
  [Lq_over_LB_AXI] -> Product3/2  "Lq_over_LB"
  [omega_m_pu] -> Product4/1  "omega_m_pu"
  [polepairs_AXI] -> Product4/2  "polepairs"
  [Ts_times_ZB_over_Lq_AXI] -> Product5/1  "Ts_times_ZB_over_Lq"
  [iq_pu] -> Product6/2  "iq_k_pu"
  [Rs_over_ZB_AXI] -> Product6/1  "Rs_over_ZB"
  Add2/1 -> Product5/2
  [omega_m_pu] -> Product9/1  "omega_m_pu"
  [iq_pu] -> Add3/2  "iq_k_pu"
  [id_pu] -> Product8/1  "id_k_pu"
  [Ld_over_LB_AXI] -> Product8/2  "Ld_over_LB"
  [polepairs_AXI] -> Product9/2  "polepairs"
  Product5/1 -> Add3/1
  [psi_pm_over_psiB_AXI] -> Product10/1
  [Ts_times_ZB_over_Lx_AXI] -> Product11/1  "Ts_times_ZB_over_Lx"
  [ix_pu] -> Product12/2  "ix_k_pu"
  [Rs_over_ZB_AXI] -> Product12/1  "Rs_over_ZB"
  Add4/1 -> Product11/2
  [ix_pu] -> Add5/2  "ix_k_pu"
  Product11/1 -> Add5/1
  [Rs_over_ZB_AXI] -> Product14/1  "Rs_over_ZB"
  Add6/1 -> Product13/2
  [iy_pu] -> Add7/2  "iy_k_pu"
  [iy_pu] -> Product14/2  "iy_k_pu"
  [Ts_times_ZB_over_Ly_AXI] -> Product13/1  "Ts_times_ZB_over_Ly"
  Product13/1 -> Add7/1
  Product2/1 -> Delay1/1
  Product1/1 -> Delay10/1
  Delay10/1 -> Add/2
  Delay1/1 -> Add/3
  [vd_pu] -> Delay18/1  "vd_pu"
  Delay18/1 -> Add/1
  [vq_pu] -> Delay19/1  "vq_pu"
  Product7/1 -> Delay21/1
  Product10/1 -> Delay22/1
  Delay22/1 -> Add2/4
  Delay21/1 -> Add2/3
  Delay20/1 -> Add2/2
  Delay19/1 -> Add2/1
  Product6/1 -> Delay20/1
  [vx_pu] -> Delay23/1  "vx_pu"
  Delay23/1 -> Add4/1
  Product12/1 -> Delay24/1
  Delay24/1 -> Add4/2
  [vy_pu] -> Delay41/1  "vy_pu"
  Product14/1 -> Delay42/1
  Delay42/1 -> Add6/2
  Delay41/1 -> Add6/1
  Product4/1 -> Delay45/1
  Product3/1 -> Delay46/1
  Delay46/1 -> Product2/2
  Delay45/1 -> Product2/1
  Product9/1 -> Delay47/1
  Delay47/1 -> Product10/2, Product7/1
  Product8/1 -> Delay48/1
  Delay48/1 -> Product7/2
  Detect Rise Positive1/1 -> Delay11/1, Switch31/2, Switch30/2, Switch29/2, Scope/3, Switch28/2  "delay_comp done"
  trigger_prediction/1 -> Delay50/1
  Delay50/1 -> Detect Rise Positive1/1
  Detect Rise Positive/1 -> Switch21/2, Switch19/2, Switch18/2, Switch17/2, Switch16/2, Switch15/2, Switch14/2, Switch13/2, Switch12/2, Switch5/2, Switch3/2, Switch2/2, Switch1/2, Scope/4, Switch/2

== system uz_mpc_6ph_sca/pu_omega_m ==
  in1 : Inport  OutDataTypeStr=fixdt(1,24,11)
  AXI_pu_conv_in : Inport  Port=2  OutDataTypeStr=fixdt(0,18,18)
  adc_valid_trigger : Inport  Port=3  OutDataTypeStr=boolean
  Delay{32,64,127..129} (5 alike) : Delay
  Delay31 : Delay  DelayLength=1
  Detect Rise Positive : simulink/Logic and Bit Operations/Detect Rise Positive  vinit=0  OutDataTypeStr=boolean
  Product23 : Product  OutDataTypeStr=fixdt(1,24,11)
  Switch31 : Switch  Criteria=u2 > Threshold  SaturateOnIntegerOverflow=off  InputSameDT=off
  out1 : Outport
  pu_conv_done : Outport  Port=2  OutDataTypeStr=boolean  LockScale=on
  out1_AXI : Outport  Port=3
  wires:
  adc_valid_trigger/1 -> Delay32/1
  in1/1 -> Delay64/1
  Delay129/1 -> pu_conv_done/1
  AXI_pu_conv_in/1 -> Product23/1
  Delay64/1 -> Switch31/1
  Delay128/1 -> out1_AXI/1
  Delay32/1 -> Detect Rise Positive/1
  Switch31/1 -> Product23/2, Delay31/1
  Delay31/1 -> Switch31/3
  Detect Rise Positive/1 -> Delay129/1, Switch31/2
  Product23/1 -> Delay127/1, Delay128/1
  Delay127/1 -> out1/1

== system uz_mpc_6ph_sca/pu_omega_m1 ==
  in1 : Inport  OutDataTypeStr=fixdt(1,24,11)
  AXI_pu_conv_in : Inport  Port=2  OutDataTypeStr=fixdt(0,18,18)
  adc_valid_trigger : Inport  Port=3  OutDataTypeStr=boolean
  Delay{32,64,127..129} (5 alike) : Delay
  Delay31 : Delay  DelayLength=1
  Detect Rise Positive : simulink/Logic and Bit Operations/Detect Rise Positive  vinit=0  OutDataTypeStr=boolean
  Product23 : Product  OutDataTypeStr=fixdt(1,24,11)
  Switch31 : Switch  Criteria=u2 > Threshold  SaturateOnIntegerOverflow=off  InputSameDT=off
  out1 : Outport
  pu_conv_done : Outport  Port=2  OutDataTypeStr=boolean  LockScale=on
  out1_AXI : Outport  Port=3
  wires:
  adc_valid_trigger/1 -> Delay32/1
  in1/1 -> Delay64/1
  Delay129/1 -> pu_conv_done/1
  AXI_pu_conv_in/1 -> Product23/1
  Delay64/1 -> Switch31/1
  Delay128/1 -> out1_AXI/1
  Delay32/1 -> Detect Rise Positive/1
  Switch31/1 -> Product23/2, Delay31/1
  Delay31/1 -> Switch31/3
  Detect Rise Positive/1 -> Delay129/1, Switch31/2
  Product23/1 -> Delay127/1, Delay128/1
  Delay127/1 -> out1/1
